simulink library "EstebanPowerLIB"  (R2013a)
settings: Solver=ode45  StartTime=0.0  StopTime=10.0  RelTol=1e-3
libraries: fl_lib x64, nesl_utility x31, elec_lib x6, dsparch4 x1
settings Model: Creator=Esteban  LastModifiedBy=Esteban

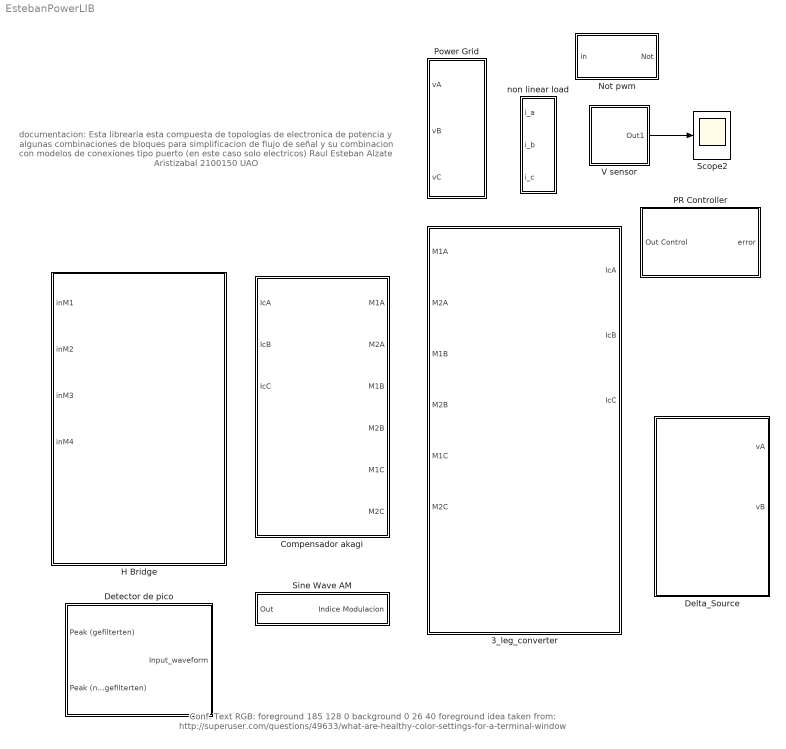
== system EstebanPowerLIB ==
  note: documentacion:
      |
      |
      | Esta librearia esta compuesta
      | de topologias de electronica de potencia
      | y algunas combinaciones de bloques
      | para simplificacion de flujo de señal
      | y su combinacion con modelos de conexiones
      | tipo puerto (en este caso solo electricos)
      |
      | Raul Esteban Alzate Aristizabal 2100150 UAO
  note: Conf. Text
      | RGB:
      | foreground 185 128 0
      | background 0 26 40
      | foreground idea taken from:
      | http://superuser.com/questions/49633/what-are-healthy-color-settings-for-a-terminal-window
  3_leg_converter : Subsystem
  Compensador akagi : Subsystem
  Delta_Source : Subsystem
  Detector de pico : Subsystem
  H Bridge : Subsystem
  Not pwm : Subsystem
  PR Controller : Subsystem
  Power Grid : Subsystem
  Scope2 : Scope
  Sine Wave AM : Subsystem
  V sensor : Subsystem
  non linear load : Subsystem
  wires:
  V sensor/1(Out1) -> Scope2/1

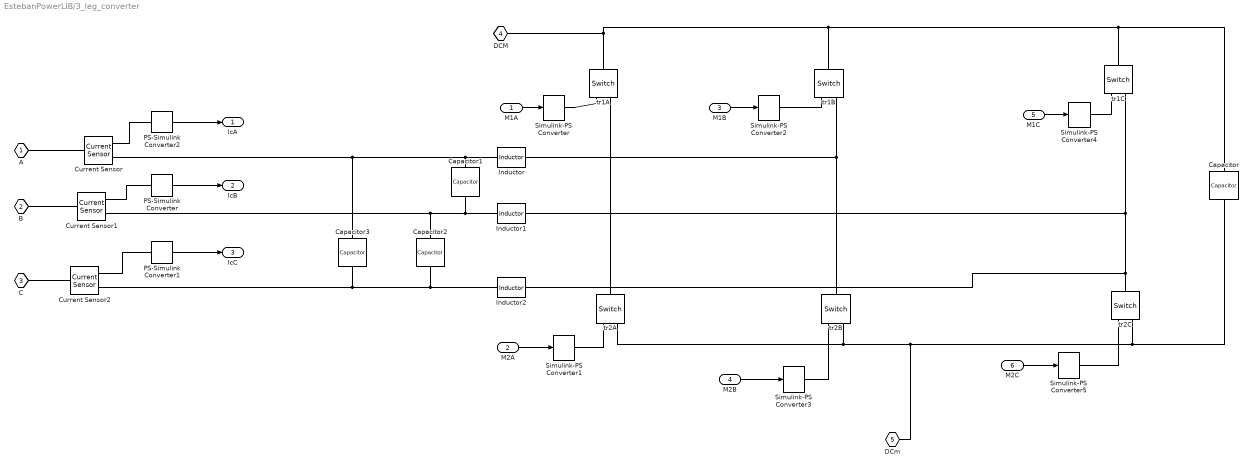
== system EstebanPowerLIB/3_leg_converter ==
  M1A : Inport
  M2A : Inport  Port=2
  M1B : Inport  Port=3
  M2B : Inport  Port=4
  M1C : Inport  Port=5
  M2C : Inport  Port=6
  Capacitor : fl_lib/Electrical/Electrical Elements/Capacitor  c=5 uF  v0=0 V  r=1e-6 Ohm  g=0 1/Ohm  i_Log=off  v_Log=off  vc_Log=off  LocalVarNames=|i|v|vc  LocalVarDescs=|i|v|Internal variable for voltage across capacitor term  LocalVarLogging=[0 0 0]
  Capacitor1 : fl_lib/Electrical/Electrical Elements/Capacitor  c=0.5 uF  v0=0 V  r=1e-6 Ohm  g=13e-8 1/Ohm  i_Log=off  v_Log=off  vc_Log=off  LocalVarNames=|i|v|vc  LocalVarDescs=|i|v|Internal variable for voltage across capacitor term  LocalVarLogging=[0 0 0]
  Capacitor2 : fl_lib/Electrical/Electrical Elements/Capacitor  c=0.5 uF  v0=0 V  r=1e-6 Ohm  g=13e-8 1/Ohm  i_Log=off  v_Log=off  vc_Log=off  LocalVarNames=|i|v|vc  LocalVarDescs=|i|v|Internal variable for voltage across capacitor term  LocalVarLogging=[0 0 0]
  Capacitor3 : fl_lib/Electrical/Electrical Elements/Capacitor  c=0.5 uF  v0=0 V  r=1e-6 Ohm  g=13e-8 1/Ohm  i_Log=off  v_Log=off  vc_Log=off  LocalVarNames=|i|v|vc  LocalVarDescs=|i|v|Internal variable for voltage across capacitor term  LocalVarLogging=[0 0 0]
  Current Sensor : fl_lib/Electrical/Electrical Sensors/Current Sensor  i1_Log=off  v1_Log=off  LocalVarNames=|i1|v1  LocalVarDescs=|i1|v1  LocalVarLogging=[0 0]
  Current Sensor1 : fl_lib/Electrical/Electrical Sensors/Current Sensor  i1_Log=off  v1_Log=off  LocalVarNames=|i1|v1  LocalVarDescs=|i1|v1  LocalVarLogging=[0 0]
  Current Sensor2 : fl_lib/Electrical/Electrical Sensors/Current Sensor  i1_Log=off  v1_Log=off  LocalVarNames=|i1|v1  LocalVarDescs=|i1|v1  LocalVarLogging=[0 0]
  Inductor : fl_lib/Electrical/Electrical Elements/Inductor  l=2.4 mH  i0=0 A  r=0.1 Ohm  g=1e-5 1/Ohm  i_Log=off  v_Log=off  i_L_Log=off  LocalVarNames=|i|v|i_L  LocalVarDescs=|i|v|Internal variable for current through inductor term  LocalVarLogging=[0 0 0]
  Inductor1 : fl_lib/Electrical/Electrical Elements/Inductor  l=2.4 mH  i0=0 A  r=0.1 Ohm  g=1e-5 1/Ohm  i_Log=off  v_Log=off  i_L_Log=off  LocalVarNames=|i|v|i_L  LocalVarDescs=|i|v|Internal variable for current through inductor term  LocalVarLogging=[0 0 0]
  Inductor2 : fl_lib/Electrical/Electrical Elements/Inductor  l=2.4 mH  i0=0 A  r=0.1 Ohm  g=1e-5 1/Ohm  i_Log=off  v_Log=off  i_L_Log=off  LocalVarNames=|i|v|i_L  LocalVarDescs=|i|v|Internal variable for current through inductor term  LocalVarLogging=[0 0 0]
  PS-Simulink Converter : nesl_utility/PS-Simulink Converter  PhysicalDomain=network_engine_domain  SubClassName=ps_output  LeftPortType=input  RightPortType=output  PseudoPeriodic=off  Frequencies=[]  Unit=1  AffineConversion=off
  PS-Simulink Converter1 : nesl_utility/PS-Simulink Converter  PhysicalDomain=network_engine_domain  SubClassName=ps_output  LeftPortType=input  RightPortType=output  PseudoPeriodic=off  Frequencies=[]  Unit=1  AffineConversion=off
  PS-Simulink Converter2 : nesl_utility/PS-Simulink Converter  PhysicalDomain=network_engine_domain  SubClassName=ps_output  LeftPortType=input  RightPortType=output  PseudoPeriodic=off  Frequencies=[]  Unit=1  AffineConversion=off
  Simulink-PS Converter{,1..5} (6 alike) : nesl_utility/Simulink-PS Converter  PhysicalDomain=network_engine_domain  SubClassName=ps_input  LeftPortType=input  RightPortType=output  PseudoPeriodic=off  Frequencies=[]  NoiseDistribution=none  NoiseParameters=[]  Unit=1  AffineConversion=off  InputFiltering=off  SimscapeFilterOrder=1  InputFilterTimeConstant=0.001  UdotUserProvided=1
  tr1A : fl_lib/Electrical/Electrical Elements/Switch  R_closed=0.01 Ohm  G_open=1e-8 1/Ohm  Threshold=10  i_Log=off  v_Log=off  LocalVarNames=|i|v  LocalVarDescs=|i|v  LocalVarLogging=[0 0]
  tr1B : fl_lib/Electrical/Electrical Elements/Switch  R_closed=0.01 Ohm  G_open=1e-8 1/Ohm  Threshold=10  i_Log=off  v_Log=off  LocalVarNames=|i|v  LocalVarDescs=|i|v  LocalVarLogging=[0 0]
  tr1C : fl_lib/Electrical/Electrical Elements/Switch  R_closed=0.01 Ohm  G_open=1e-8 1/Ohm  Threshold=10  i_Log=off  v_Log=off  LocalVarNames=|i|v  LocalVarDescs=|i|v  LocalVarLogging=[0 0]
  tr2A : fl_lib/Electrical/Electrical Elements/Switch  R_closed=0.01 Ohm  G_open=1e-8 1/Ohm  Threshold=10  i_Log=off  v_Log=off  LocalVarNames=|i|v  LocalVarDescs=|i|v  LocalVarLogging=[0 0]
  tr2B : fl_lib/Electrical/Electrical Elements/Switch  R_closed=0.01 Ohm  G_open=1e-8 1/Ohm  Threshold=10  i_Log=off  v_Log=off  LocalVarNames=|i|v  LocalVarDescs=|i|v  LocalVarLogging=[0 0]
  tr2C : fl_lib/Electrical/Electrical Elements/Switch  R_closed=0.01 Ohm  G_open=1e-8 1/Ohm  Threshold=10  i_Log=off  v_Log=off  LocalVarNames=|i|v  LocalVarDescs=|i|v  LocalVarLogging=[0 0]
  A : PMIOPort  Port=1  Side=Right
  B : PMIOPort  Port=2  Side=Right
  C : PMIOPort  Port=3  Side=Right
  DCM : PMIOPort  Port=4  Side=Left
  DCm : PMIOPort  Port=5  Side=Left
  IcA : Outport
  IcB : Outport  Port=2
  IcC : Outport  Port=3
  wires:
  M2C/1 -> Simulink-PS Converter5/1
  M1C/1 -> Simulink-PS Converter4/1
  M2B/1 -> Simulink-PS Converter3/1
  M1B/1 -> Simulink-PS Converter2/1
  M2A/1 -> Simulink-PS Converter1/1
  M1A/1 -> Simulink-PS Converter/1
  PS-Simulink Converter2/1 -> IcA/1
  PS-Simulink Converter/1 -> IcB/1
  PS-Simulink Converter1/1 -> IcC/1
  connections:
  Simulink-PS Converter3/RConn1 -- tr2B/RConn1
  Simulink-PS Converter4/RConn1 -- tr1C/RConn1
  Simulink-PS Converter/RConn1 -- tr1A/RConn1
  Simulink-PS Converter5/RConn1 -- tr2C/RConn1
  tr2A/RConn1 -- Simulink-PS Converter1/RConn1
  tr2C/RConn2 -- DCm/RConn1 -- tr2A/RConn2 -- tr2B/RConn2 -- Capacitor/RConn1
  tr1A/RConn2 -- tr2A/LConn1
  tr1B/RConn2 -- Inductor/RConn1 -- tr2B/LConn1
  Capacitor/LConn1 -- tr1C/LConn1 -- DCM/RConn1 -- tr1A/LConn1 -- tr1B/LConn1
  tr1C/RConn2 -- Inductor1/RConn1 -- Inductor2/RConn1 -- tr2C/LConn1
  tr1B/RConn1 -- Simulink-PS Converter2/RConn1
  Capacitor1/LConn1 -- Inductor/LConn1 -- Capacitor3/LConn1 -- Current Sensor/RConn2
  Capacitor1/RConn1 -- Inductor1/LConn1 -- Capacitor2/LConn1 -- Current Sensor1/RConn2
  Capacitor2/RConn1 -- Inductor2/LConn1 -- Current Sensor2/RConn2 -- Capacitor3/RConn1
  Current Sensor1/RConn1 -- PS-Simulink Converter/LConn1
  Current Sensor/RConn1 -- PS-Simulink Converter2/LConn1
  Current Sensor2/RConn1 -- PS-Simulink Converter1/LConn1
  B/RConn1 -- Current Sensor1/LConn1
  A/RConn1 -- Current Sensor/LConn1
  Current Sensor2/LConn1 -- C/RConn1

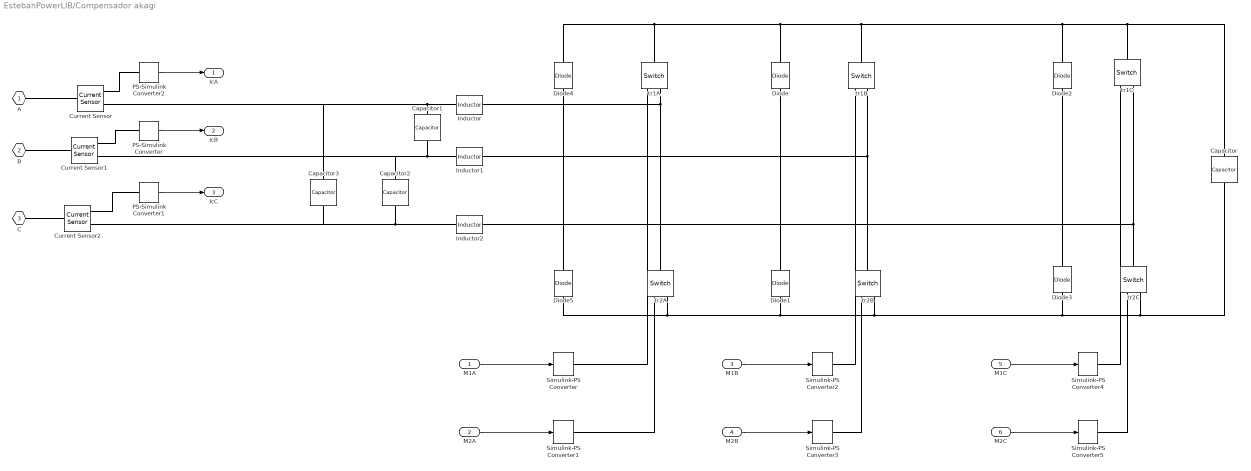
== system EstebanPowerLIB/Compensador akagi ==
  M1A : Inport
  M2A : Inport  Port=2
  M1B : Inport  Port=3
  M2B : Inport  Port=4
  M1C : Inport  Port=5
  M2C : Inport  Port=6
  Capacitor : fl_lib/Electrical/Electrical Elements/Capacitor  c=5 uF  v0=0 V  r=1e-6 Ohm  g=0 1/Ohm  i_Log=off  v_Log=off  vc_Log=off  LocalVarNames=|i|v|vc  LocalVarDescs=|i|v|Internal variable for voltage across capacitor term  LocalVarLogging=[0 0 0]
  Capacitor1 : fl_lib/Electrical/Electrical Elements/Capacitor  c=0.5 uF  v0=0 V  r=1e-6 Ohm  g=0 1/Ohm  i_Log=off  v_Log=off  vc_Log=off  LocalVarNames=|i|v|vc  LocalVarDescs=|i|v|Internal variable for voltage across capacitor term  LocalVarLogging=[0 0 0]
  Capacitor2 : fl_lib/Electrical/Electrical Elements/Capacitor  c=0.5 uF  v0=0 V  r=1e-6 Ohm  g=0 1/Ohm  i_Log=off  v_Log=off  vc_Log=off  LocalVarNames=|i|v|vc  LocalVarDescs=|i|v|Internal variable for voltage across capacitor term  LocalVarLogging=[0 0 0]
  Capacitor3 : fl_lib/Electrical/Electrical Elements/Capacitor  c=0.5 uF  v0=0 V  r=1e-6 Ohm  g=0 1/Ohm  i_Log=off  v_Log=off  vc_Log=off  LocalVarNames=|i|v|vc  LocalVarDescs=|i|v|Internal variable for voltage across capacitor term  LocalVarLogging=[0 0 0]
  Current Sensor : fl_lib/Electrical/Electrical Sensors/Current Sensor  i1_Log=off  v1_Log=off  LocalVarNames=|i1|v1  LocalVarDescs=|i1|v1  LocalVarLogging=[0 0]
  Current Sensor1 : fl_lib/Electrical/Electrical Sensors/Current Sensor  i1_Log=off  v1_Log=off  LocalVarNames=|i1|v1  LocalVarDescs=|i1|v1  LocalVarLogging=[0 0]
  Current Sensor2 : fl_lib/Electrical/Electrical Sensors/Current Sensor  i1_Log=off  v1_Log=off  LocalVarNames=|i1|v1  LocalVarDescs=|i1|v1  LocalVarLogging=[0 0]
  Diode{,1..5} (6 alike) : fl_lib/Electrical/Electrical Elements/Diode  Vf=0.6 V  Ron=0.3 Ohm  Goff=1e-8 1/Ohm  i_Log=off  v_Log=off  LocalVarNames=|i|v  LocalVarDescs=|i|v  LocalVarLogging=[0 0]
  Inductor : fl_lib/Electrical/Electrical Elements/Inductor  l=2.4 mH  i0=0 A  r=0.1 Ohm  g=1e-9 1/Ohm  i_Log=off  v_Log=off  i_L_Log=off  LocalVarNames=|i|v|i_L  LocalVarDescs=|i|v|Internal variable for current through inductor term  LocalVarLogging=[0 0 0]
  Inductor1 : fl_lib/Electrical/Electrical Elements/Inductor  l=2.4 mH  i0=0 A  r=0.1 Ohm  g=1e-9 1/Ohm  i_Log=off  v_Log=off  i_L_Log=off  LocalVarNames=|i|v|i_L  LocalVarDescs=|i|v|Internal variable for current through inductor term  LocalVarLogging=[0 0 0]
  Inductor2 : fl_lib/Electrical/Electrical Elements/Inductor  l=2.4 mH  i0=0 A  r=0.1 Ohm  g=1e-9 1/Ohm  i_Log=off  v_Log=off  i_L_Log=off  LocalVarNames=|i|v|i_L  LocalVarDescs=|i|v|Internal variable for current through inductor term  LocalVarLogging=[0 0 0]
  PS-Simulink Converter : nesl_utility/PS-Simulink Converter  PhysicalDomain=network_engine_domain  SubClassName=ps_output  LeftPortType=input  RightPortType=output  PseudoPeriodic=off  Frequencies=[]  Unit=1  AffineConversion=off
  PS-Simulink Converter1 : nesl_utility/PS-Simulink Converter  PhysicalDomain=network_engine_domain  SubClassName=ps_output  LeftPortType=input  RightPortType=output  PseudoPeriodic=off  Frequencies=[]  Unit=1  AffineConversion=off
  PS-Simulink Converter2 : nesl_utility/PS-Simulink Converter  PhysicalDomain=network_engine_domain  SubClassName=ps_output  LeftPortType=input  RightPortType=output  PseudoPeriodic=off  Frequencies=[]  Unit=1  AffineConversion=off
  Simulink-PS Converter{,1..5} (6 alike) : nesl_utility/Simulink-PS Converter  PhysicalDomain=network_engine_domain  SubClassName=ps_input  LeftPortType=input  RightPortType=output  PseudoPeriodic=off  Frequencies=[]  NoiseDistribution=none  NoiseParameters=[]  Unit=1  AffineConversion=off  InputFiltering=off  SimscapeFilterOrder=1  InputFilterTimeConstant=0.001  UdotUserProvided=1
  tr1A : fl_lib/Electrical/Electrical Elements/Switch  R_closed=0.01 Ohm  G_open=1e-8 1/Ohm  Threshold=10  i_Log=off  v_Log=off  LocalVarNames=|i|v  LocalVarDescs=|i|v  LocalVarLogging=[0 0]
  tr1B : fl_lib/Electrical/Electrical Elements/Switch  R_closed=0.01 Ohm  G_open=1e-8 1/Ohm  Threshold=10  i_Log=off  v_Log=off  LocalVarNames=|i|v  LocalVarDescs=|i|v  LocalVarLogging=[0 0]
  tr1C : fl_lib/Electrical/Electrical Elements/Switch  R_closed=0.01 Ohm  G_open=1e-8 1/Ohm  Threshold=10  i_Log=off  v_Log=off  LocalVarNames=|i|v  LocalVarDescs=|i|v  LocalVarLogging=[0 0]
  tr2A : fl_lib/Electrical/Electrical Elements/Switch  R_closed=0.01 Ohm  G_open=1e-8 1/Ohm  Threshold=10  i_Log=off  v_Log=off  LocalVarNames=|i|v  LocalVarDescs=|i|v  LocalVarLogging=[0 0]
  tr2B : fl_lib/Electrical/Electrical Elements/Switch  R_closed=0.01 Ohm  G_open=1e-8 1/Ohm  Threshold=10  i_Log=off  v_Log=off  LocalVarNames=|i|v  LocalVarDescs=|i|v  LocalVarLogging=[0 0]
  tr2C : fl_lib/Electrical/Electrical Elements/Switch  R_closed=0.01 Ohm  G_open=1e-8 1/Ohm  Threshold=10  i_Log=off  v_Log=off  LocalVarNames=|i|v  LocalVarDescs=|i|v  LocalVarLogging=[0 0]
  A : PMIOPort  Port=1  Side=Right
  B : PMIOPort  Port=2  Side=Right
  C : PMIOPort  Port=3  Side=Right
  IcA : Outport
  IcB : Outport  Port=2
  IcC : Outport  Port=3
  wires:
  M1A/1 -> Simulink-PS Converter/1
  M2A/1 -> Simulink-PS Converter1/1
  M1B/1 -> Simulink-PS Converter2/1
  M2B/1 -> Simulink-PS Converter3/1
  M1C/1 -> Simulink-PS Converter4/1
  M2C/1 -> Simulink-PS Converter5/1
  PS-Simulink Converter2/1 -> IcA/1
  PS-Simulink Converter/1 -> IcB/1
  PS-Simulink Converter1/1 -> IcC/1
  connections:
  tr2A/RConn2 -- Diode1/LConn1 -- tr2B/RConn2 -- Diode3/LConn1 -- Capacitor/RConn1 -- tr2C/RConn2 -- Diode5/LConn1
  tr1A/RConn2 -- tr2A/LConn1 -- Inductor/RConn1 -- Diode5/RConn1 -- Diode4/LConn1
  tr1B/RConn2 -- Inductor1/RConn1 -- Diode/LConn1 -- Diode1/RConn1 -- tr2B/LConn1
  tr1C/LConn1 -- Diode2/RConn1 -- Diode/RConn1 -- Diode4/RConn1 -- tr1A/LConn1 -- tr1B/LConn1 -- Capacitor/LConn1
  tr1C/RConn2 -- Inductor2/RConn1 -- Diode3/RConn1 -- Diode2/LConn1 -- tr2C/LConn1
  Inductor/LConn1 -- Capacitor3/LConn1 -- Current Sensor/RConn2 -- Capacitor1/LConn1
  Inductor1/LConn1 -- Capacitor2/LConn1 -- Current Sensor1/RConn2 -- Capacitor1/RConn1
  Inductor2/LConn1 -- Current Sensor2/RConn2 -- Capacitor3/RConn1 -- Capacitor2/RConn1
  Simulink-PS Converter/RConn1 -- tr1A/RConn1
  Simulink-PS Converter1/RConn1 -- tr2A/RConn1
  Simulink-PS Converter3/RConn1 -- tr2B/RConn1
  Simulink-PS Converter2/RConn1 -- tr1B/RConn1
  Simulink-PS Converter4/RConn1 -- tr1C/RConn1
  Simulink-PS Converter5/RConn1 -- tr2C/RConn1
  A/RConn1 -- Current Sensor/LConn1
  B/RConn1 -- Current Sensor1/LConn1
  Current Sensor2/LConn1 -- C/RConn1
  Current Sensor2/RConn1 -- PS-Simulink Converter1/LConn1
  Current Sensor1/RConn1 -- PS-Simulink Converter/LConn1
  Current Sensor/RConn1 -- PS-Simulink Converter2/LConn1

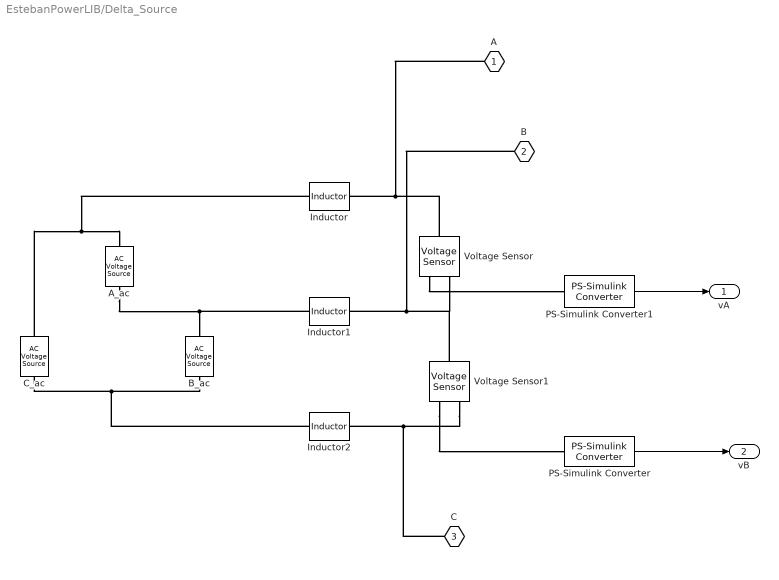
== system EstebanPowerLIB/Delta_Source ==
  A_ac : fl_lib/Electrical/Electrical Sources/AC Voltage Source  amp=170 V  shift=0 deg  frequency=60 Hz  omega=0 rad/s  i_Log=off  v_Log=off  LocalVarNames=|i|v  LocalVarDescs=|i|v  LocalVarLogging=[0 0]
  B_ac : fl_lib/Electrical/Electrical Sources/AC Voltage Source  amp=170 V  shift=-120 deg  frequency=60 Hz  omega=0 rad/s  i_Log=off  v_Log=off  LocalVarNames=|i|v  LocalVarDescs=|i|v  LocalVarLogging=[0 0]
  C_ac : fl_lib/Electrical/Electrical Sources/AC Voltage Source  amp=170 V  shift=120 deg  frequency=60 Hz  omega=0 rad/s  i_Log=off  v_Log=off  LocalVarNames=|i|v  LocalVarDescs=|i|v  LocalVarLogging=[0 0]
  Inductor : fl_lib/Electrical/Electrical Elements/Inductor  l=2 mH  i0=0 A  r=0.2 Ohm  g=1e-4 1/Ohm  i_Log=off  v_Log=off  i_L_Log=off  LocalVarNames=|i|v|i_L  LocalVarDescs=|i|v|Internal variable for current through inductor term  LocalVarLogging=[0 0 0]
  Inductor1 : fl_lib/Electrical/Electrical Elements/Inductor  l=2 mH  i0=0 A  r=0.2 Ohm  g=1e-4 1/Ohm  i_Log=off  v_Log=off  i_L_Log=off  LocalVarNames=|i|v|i_L  LocalVarDescs=|i|v|Internal variable for current through inductor term  LocalVarLogging=[0 0 0]
  Inductor2 : fl_lib/Electrical/Electrical Elements/Inductor  l=2 mH  i0=0 A  r=0.1 Ohm  g=1e-4 1/Ohm  i_Log=off  v_Log=off  i_L_Log=off  LocalVarNames=|i|v|i_L  LocalVarDescs=|i|v|Internal variable for current through inductor term  LocalVarLogging=[0 0 0]
  PS-Simulink Converter : nesl_utility/PS-Simulink Converter  PhysicalDomain=network_engine_domain  SubClassName=ps_output  LeftPortType=input  RightPortType=output  PseudoPeriodic=off  Frequencies=[]  Unit=1  AffineConversion=off
  PS-Simulink Converter1 : nesl_utility/PS-Simulink Converter  PhysicalDomain=network_engine_domain  SubClassName=ps_output  LeftPortType=input  RightPortType=output  PseudoPeriodic=off  Frequencies=[]  Unit=1  AffineConversion=off
  Voltage Sensor : fl_lib/Electrical/Electrical Sensors/Voltage Sensor  i1_Log=off  v1_Log=off  LocalVarNames=|i1|v1  LocalVarDescs=|i1|v1  LocalVarLogging=[0 0]
  Voltage Sensor1 : fl_lib/Electrical/Electrical Sensors/Voltage Sensor  i1_Log=off  v1_Log=off  LocalVarNames=|i1|v1  LocalVarDescs=|i1|v1  LocalVarLogging=[0 0]
  A : PMIOPort  Port=1  Side=Left
  B : PMIOPort  Port=2  Side=Right
  C : PMIOPort  Port=3  Side=Left
  vA : Outport
  vB : Outport  Port=2
  wires:
  PS-Simulink Converter1/1 -> vA/1
  PS-Simulink Converter/1 -> vB/1
  connections:
  Voltage Sensor/RConn1 -- PS-Simulink Converter1/LConn1
  Inductor2/LConn1 -- B_ac/RConn1 -- C_ac/RConn1
  Voltage Sensor1/RConn1 -- PS-Simulink Converter/LConn1
  C/RConn1 -- Voltage Sensor1/RConn2 -- Inductor2/RConn1
  Inductor1/LConn1 -- A_ac/RConn1 -- B_ac/LConn1
  A/RConn1 -- Voltage Sensor/LConn1 -- Inductor/RConn1
  Inductor/LConn1 -- C_ac/LConn1 -- A_ac/LConn1
  B/RConn1 -- Voltage Sensor1/LConn1 -- Voltage Sensor/RConn2 -- Inductor1/RConn1

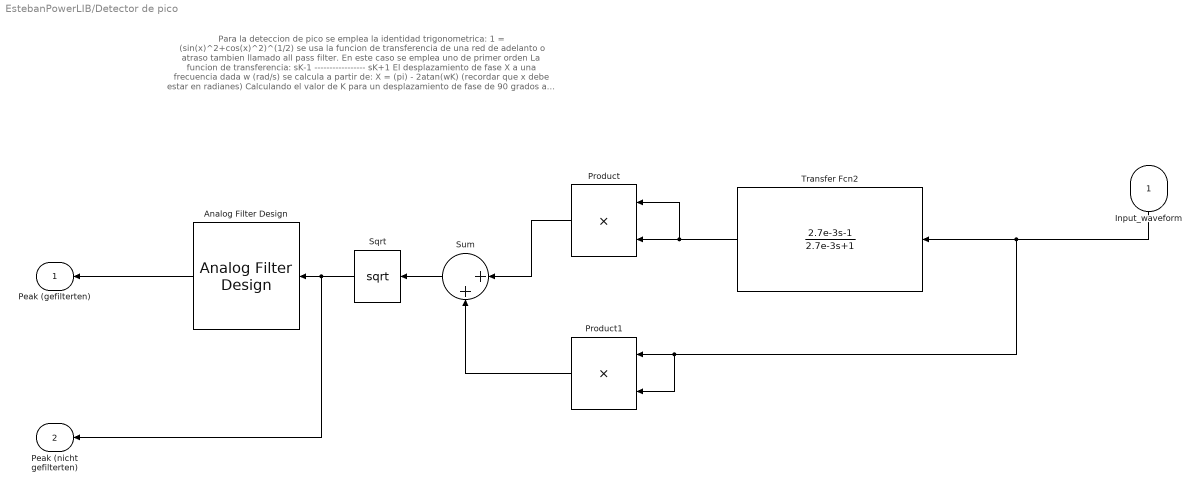
== system EstebanPowerLIB/Detector de pico ==
  note: Para la deteccion de pico se emplea la identidad trigonometrica:
      | 1 = (sin(x)^2+cos(x)^2)^(1/2)
      | se usa la funcion de transferencia de una red de adelanto o atraso
      | tambien llamado all pass filter. En este caso se emplea uno de primer orden
      | La funcion de transferencia:
      | sK-1
      | -----------------
      | sK+1
      | El desplazamiento de fase X a una frecuencia dada w (rad/s) se calcula a partir de:
      | X = (pi) - 2atan(wK)
      | (recordar que x debe estar en radianes)
      | Calculando el valor de K para un desplazamiento de fase de 90 grados
      | a 60 Hz se logra obtener de la señal su "coseno".
      | seguido de esto solo basta con elevarlas ambas al cuadrado y sumarlas.
      | finalmente la raiz cuadrada es el valor pico de la señal y este metodo es aplicable durante
      | todo el periodo de la forma de onda. para reducir el ruido por conmutacion se agrega un  filtro
      | a la salida del detector. este filtro efectivamente permite obtener una señal mas limpia
      | pero reduce la velocidad de reaccion del detector de pico. Asi como esta configurado se puede
      | esperar una desviacion de no mas que 1ms.
  Input_waveform : Inport
  Analog Filter Design : dsparch4/Analog Filter Design  method=Bessel  filttype=Lowpass  N=8  Wlo=4900*2*pi  Whi=80  Rp=2  Rs=40
  Product : Product
  Product1 : Product
  Sqrt : Sqrt  SaturateOnIntegerOverflow=on
  Sum : Sum  Inputs=|++
  Transfer Fcn2 : TransferFcn  Numerator=[2.7e-3 -1]  Denominator=[2.7e-3 +1]
  Peak (gefilterten) : Outport
  Peak (nicht gefilterten) : Outport  Port=2
  wires:
  Transfer Fcn2/1 -> Product/2, Product/1
  Sum/1 -> Sqrt/1
  Sqrt/1 -> Analog Filter Design/1, Peak (nicht gefilterten)/1
  Product/1 -> Sum/1
  Product1/1 -> Sum/2
  Analog Filter Design/1 -> Peak (gefilterten)/1
  Input_waveform/1 -> Transfer Fcn2/1, Product1/1, Product1/2

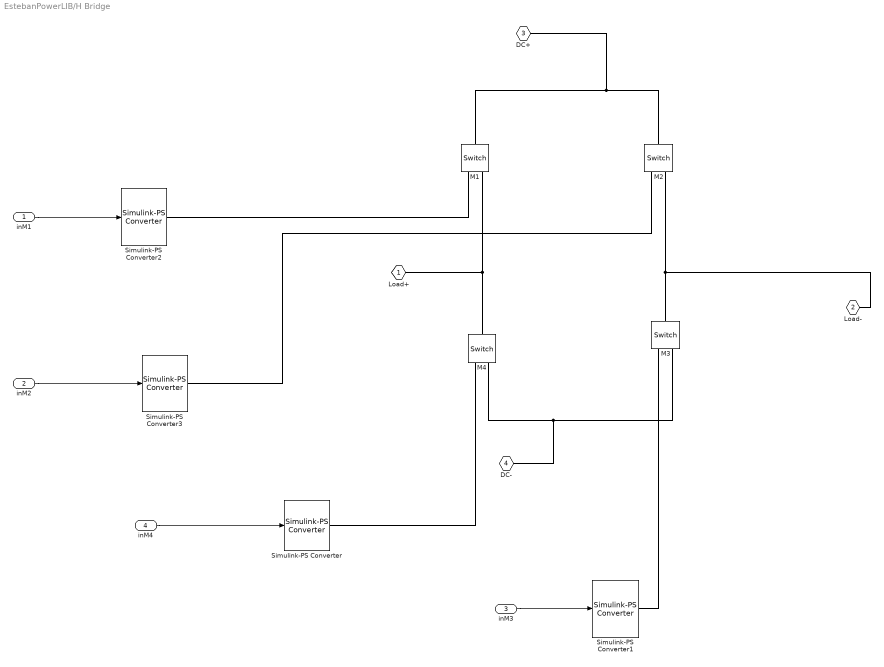
== system EstebanPowerLIB/H Bridge ==
  "inM1 " : Inport
  inM2 : Inport  Port=2
  inM3 : Inport  Port=3
  inM4 : Inport  Port=4
  M{1..4} (4 alike) : fl_lib/Electrical/Electrical Elements/Switch  R_closed=0.01 Ohm  G_open=1e-8 1/Ohm  Threshold=10  i_Log=off  v_Log=off  LocalVarNames=|i|v  LocalVarDescs=|i|v  LocalVarLogging=[0 0]
  Simulink-PS Converter{,1..3} (4 alike) : nesl_utility/Simulink-PS Converter  PhysicalDomain=network_engine_domain  SubClassName=ps_input  LeftPortType=input  RightPortType=output  PseudoPeriodic=off  Frequencies=[]  NoiseDistribution=none  NoiseParameters=[]  Unit=1  AffineConversion=off  InputFiltering=off  SimscapeFilterOrder=1  InputFilterTimeConstant=0.001  UdotUserProvided=1
  Load+ : PMIOPort  Port=1  Side=Right
  Load- : PMIOPort  Port=2  Side=Right
  DC+ : PMIOPort  Port=3  Side=Left
  DC- : PMIOPort  Port=4  Side=Left
  wires:
  "inM1 "/1 -> Simulink-PS Converter2/1
  inM2/1 -> Simulink-PS Converter3/1
  inM3/1 -> Simulink-PS Converter1/1
  inM4/1 -> Simulink-PS Converter/1
  connections:
  Simulink-PS Converter1/RConn1 -- M3/RConn1
  Simulink-PS Converter/RConn1 -- M4/RConn1
  Simulink-PS Converter3/RConn1 -- M2/RConn1
  Simulink-PS Converter2/RConn1 -- M1/RConn1
  M2/LConn1 -- DC+/RConn1 -- M1/LConn1
  M3/RConn2 -- DC-/RConn1 -- M4/RConn2
  M2/RConn2 -- M3/LConn1 -- Load-/RConn1
  M1/RConn2 -- Load+/RConn1 -- M4/LConn1

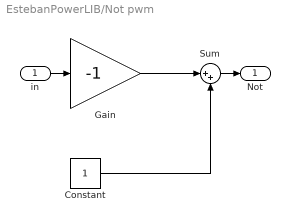
== system EstebanPowerLIB/Not pwm ==
  in : Inport
  Constant : Constant
  Gain : Gain  Gain=-1
  Sum : Sum  Inputs=|++
  Not : Outport
  wires:
  Sum/1 -> Not/1
  in/1 -> Gain/1
  Constant/1 -> Sum/2
  Gain/1 -> Sum/1

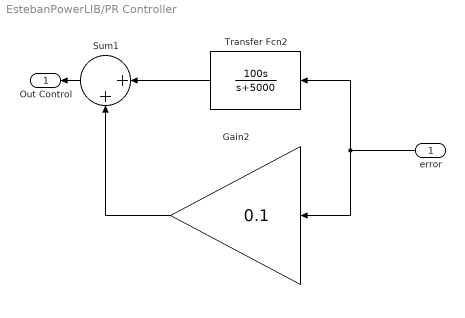
== system EstebanPowerLIB/PR Controller ==
  error : Inport
  Gain2 : Gain  Gain=0.1
  Sum1 : Sum  Inputs=|++
  Transfer Fcn2 : TransferFcn  Numerator=[100 0]  Denominator=[1 5000]
  Out Control : Outport
  wires:
  Gain2/1 -> Sum1/2
  Transfer Fcn2/1 -> Sum1/1
  Sum1/1 -> Out Control/1
  error/1 -> Transfer Fcn2/1, Gain2/1

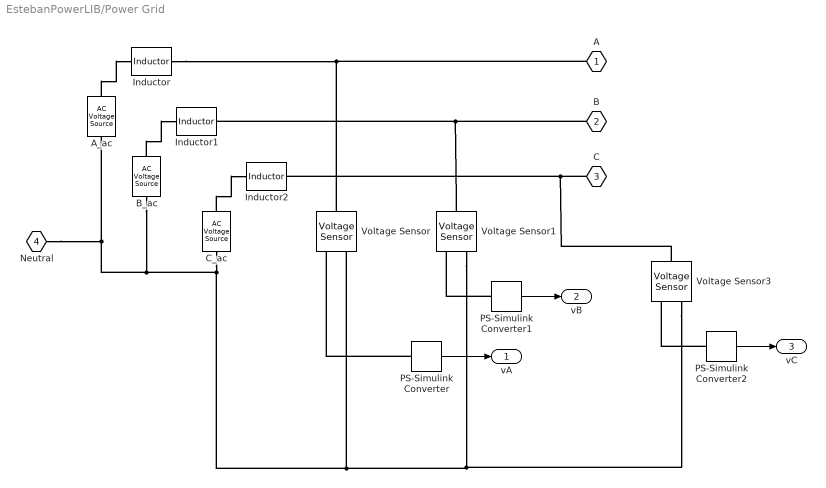
== system EstebanPowerLIB/Power Grid ==
  A_ac : fl_lib/Electrical/Electrical Sources/AC Voltage Source  amp=170 V  shift=0 deg  frequency=60 Hz  omega=0 rad/s  i_Log=off  v_Log=off  LocalVarNames=|i|v  LocalVarDescs=|i|v  LocalVarLogging=[0 0]
  B_ac : fl_lib/Electrical/Electrical Sources/AC Voltage Source  amp=170 V  shift=-120 deg  frequency=60 Hz  omega=0 rad/s  i_Log=off  v_Log=off  LocalVarNames=|i|v  LocalVarDescs=|i|v  LocalVarLogging=[0 0]
  C_ac : fl_lib/Electrical/Electrical Sources/AC Voltage Source  amp=170 V  shift=120 deg  frequency=60 Hz  omega=0 rad/s  i_Log=off  v_Log=off  LocalVarNames=|i|v  LocalVarDescs=|i|v  LocalVarLogging=[0 0]
  Inductor : fl_lib/Electrical/Electrical Elements/Inductor  l=2 mH  i0=0 A  r=0.2 Ohm  g=1e-4 1/Ohm  i_Log=off  v_Log=off  i_L_Log=off  LocalVarNames=|i|v|i_L  LocalVarDescs=|i|v|Internal variable for current through inductor term  LocalVarLogging=[0 0 0]
  Inductor1 : fl_lib/Electrical/Electrical Elements/Inductor  l=2 mH  i0=0 A  r=0.2 Ohm  g=1e-4 1/Ohm  i_Log=off  v_Log=off  i_L_Log=off  LocalVarNames=|i|v|i_L  LocalVarDescs=|i|v|Internal variable for current through inductor term  LocalVarLogging=[0 0 0]
  Inductor2 : fl_lib/Electrical/Electrical Elements/Inductor  l=2 mH  i0=0 A  r=0.1 Ohm  g=1e-4 1/Ohm  i_Log=off  v_Log=off  i_L_Log=off  LocalVarNames=|i|v|i_L  LocalVarDescs=|i|v|Internal variable for current through inductor term  LocalVarLogging=[0 0 0]
  PS-Simulink Converter : nesl_utility/PS-Simulink Converter  PhysicalDomain=network_engine_domain  SubClassName=ps_output  LeftPortType=input  RightPortType=output  PseudoPeriodic=off  Frequencies=[]  Unit=1  AffineConversion=off
  PS-Simulink Converter1 : nesl_utility/PS-Simulink Converter  PhysicalDomain=network_engine_domain  SubClassName=ps_output  LeftPortType=input  RightPortType=output  PseudoPeriodic=off  Frequencies=[]  Unit=1  AffineConversion=off
  PS-Simulink Converter2 : nesl_utility/PS-Simulink Converter  PhysicalDomain=network_engine_domain  SubClassName=ps_output  LeftPortType=input  RightPortType=output  PseudoPeriodic=off  Frequencies=[]  Unit=1  AffineConversion=off
  Voltage Sensor : fl_lib/Electrical/Electrical Sensors/Voltage Sensor  i1_Log=off  v1_Log=off  LocalVarNames=|i1|v1  LocalVarDescs=|i1|v1  LocalVarLogging=[0 0]
  Voltage Sensor1 : fl_lib/Electrical/Electrical Sensors/Voltage Sensor  i1_Log=off  v1_Log=off  LocalVarNames=|i1|v1  LocalVarDescs=|i1|v1  LocalVarLogging=[0 0]
  Voltage Sensor3 : fl_lib/Electrical/Electrical Sensors/Voltage Sensor  i1_Log=off  v1_Log=off  LocalVarNames=|i1|v1  LocalVarDescs=|i1|v1  LocalVarLogging=[0 0]
  A : PMIOPort  Port=1  Side=Left
  B : PMIOPort  Port=2  Side=Left
  C : PMIOPort  Port=3  Side=Left
  Neutral : PMIOPort  Port=4  Side=Left
  vA : Outport
  vB : Outport  Port=2
  vC : Outport  Port=3
  wires:
  PS-Simulink Converter/1 -> vA/1
  PS-Simulink Converter1/1 -> vB/1
  PS-Simulink Converter2/1 -> vC/1
  connections:
  C_ac/LConn1 -- Inductor2/LConn1
  A_ac/LConn1 -- Inductor/LConn1
  B_ac/LConn1 -- Inductor1/LConn1
  B/RConn1 -- Voltage Sensor1/LConn1 -- Inductor1/RConn1
  PS-Simulink Converter/LConn1 -- Voltage Sensor/RConn1
  C/RConn1 -- Voltage Sensor3/LConn1 -- Inductor2/RConn1
  Inductor/RConn1 -- A/RConn1 -- Voltage Sensor/LConn1
  A_ac/RConn1 -- Neutral/RConn1 -- Voltage Sensor3/RConn2 -- Voltage Sensor1/RConn2 -- Voltage Sensor/RConn2 -- C_ac/RConn1 -- B_ac/RConn1
  PS-Simulink Converter1/LConn1 -- Voltage Sensor1/RConn1
  PS-Simulink Converter2/LConn1 -- Voltage Sensor3/RConn1

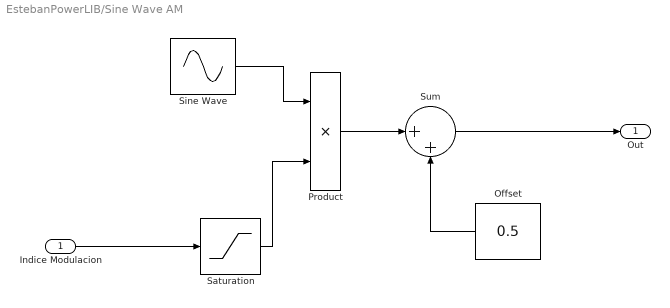
== system EstebanPowerLIB/Sine Wave AM ==
  Indice Modulacion : Inport
  Offset : Constant  Value=0.5
  Product : Product
  Saturation : Saturate  UpperLimit=1  LowerLimit=0
  Sine Wave : Sin  Amplitude=0.5  Frequency=60*2*pi  SampleTime=0
  Sum : Sum  Inputs=|++
  Out : Outport
  wires:
  Indice Modulacion/1 -> Saturation/1
  Saturation/1 -> Product/2
  Sum/1 -> Out/1
  Offset/1 -> Sum/2
  Sine Wave/1 -> Product/1
  Product/1 -> Sum/1

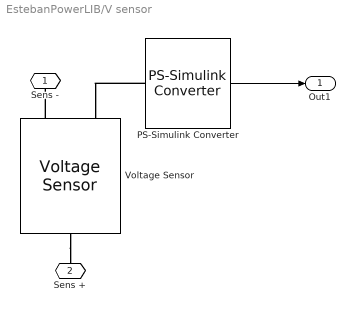
== system EstebanPowerLIB/V sensor ==
  PS-Simulink Converter : nesl_utility/PS-Simulink Converter  PhysicalDomain=network_engine_domain  SubClassName=ps_output  LeftPortType=input  RightPortType=output  PseudoPeriodic=off  Frequencies=[]  Unit=1  AffineConversion=off
  Voltage Sensor : fl_lib/Electrical/Electrical Sensors/Voltage Sensor  i1_Log=off  v1_Log=off  LocalVarNames=|i1|v1  LocalVarDescs=|i1|v1  LocalVarLogging=[0 0]
  Sens - : PMIOPort  Port=1  Side=Left
  Sens + : PMIOPort  Port=2  Side=Left
  Out1 : Outport
  wires:
  PS-Simulink Converter/1 -> Out1/1
  connections:
  Voltage Sensor/LConn1 -- Sens +/RConn1
  Voltage Sensor/RConn2 -- Sens -/RConn1
  PS-Simulink Converter/LConn1 -- Voltage Sensor/RConn1

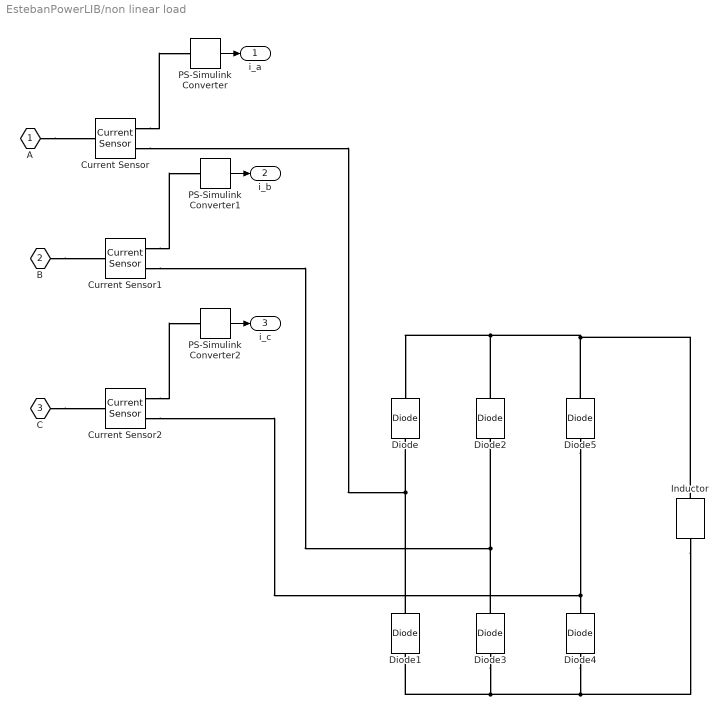
== system EstebanPowerLIB/non linear load ==
  Current Sensor : fl_lib/Electrical/Electrical Sensors/Current Sensor  i1_Log=off  v1_Log=off  LocalVarNames=|i1|v1  LocalVarDescs=|i1|v1  LocalVarLogging=[0 0]
  Current Sensor1 : fl_lib/Electrical/Electrical Sensors/Current Sensor  i1_Log=off  v1_Log=off  LocalVarNames=|i1|v1  LocalVarDescs=|i1|v1  LocalVarLogging=[0 0]
  Current Sensor2 : fl_lib/Electrical/Electrical Sensors/Current Sensor  i1_Log=off  v1_Log=off  LocalVarNames=|i1|v1  LocalVarDescs=|i1|v1  LocalVarLogging=[0 0]
  Diode{,1..5} (6 alike) : elec_lib/Semiconductor Devices/Diode  ModelType=1  Vf=0.6 V  Ron=0.3 Ohm  Goff=1e-8 S  Rz=0.3 Ohm  Vz=50 V  C_PWL=5 pF  prmExp=1  I12=[ 0.0137 0.545 ] A  V12=[ 0.6 0.7 ] V  I1=0.0137 A  V1=0.6 V  RS=0.01 Ohm  IS=1e-12 A  Tmeas=25 C  ec=1  BV=Inf V  C_param=1  CJ0=5 pF  VJ=1 V  Mgrad=0.5  Vvec=[ 0.1 10 100 ] V  Cvec=[ 3.5 1 0.4 ] pF  FC=0.5  Q_param=1  Irrm=-7.15 A  iF=4 A  didt=-750 A/us  trr=115 ns  TT=50 ns  tau=100 ns  T_param=1  IS_T2=1.25e-7 A  I1_T2=0.245 A  V1_T2=0.5 V  Tmeas2=125 C  EG_param=1  EG=1.11 eV  XTI_param=1  XTI=3  dBVdT=0 V/K  Tdevice=25 C  LocalVarLogging=[]  Rth=[ 0 10 ] K/W  thermal_mass_parameterization=1  thermal_mass=[ 0 1 ] J/K  thermal_time_constant=[ 0 10 ] s  thermal_mass_initial_temperatures=[ 25 25 ] C
  Inductor : fl_lib/Electrical/Electrical Elements/Inductor  l=2 H  i0=0 A  r=2 Ohm  g=1e-9 1/Ohm  i_Log=off  v_Log=off  i_L_Log=off  LocalVarNames=|i|v|i_L  LocalVarDescs=|i|v|Internal variable for current through inductor term  LocalVarLogging=[0 0 0]
  PS-Simulink Converter : nesl_utility/PS-Simulink Converter  PhysicalDomain=network_engine_domain  SubClassName=ps_output  LeftPortType=input  RightPortType=output  PseudoPeriodic=off  Frequencies=[]  Unit=1  AffineConversion=off
  PS-Simulink Converter1 : nesl_utility/PS-Simulink Converter  PhysicalDomain=network_engine_domain  SubClassName=ps_output  LeftPortType=input  RightPortType=output  PseudoPeriodic=off  Frequencies=[]  Unit=1  AffineConversion=off
  PS-Simulink Converter2 : nesl_utility/PS-Simulink Converter  PhysicalDomain=network_engine_domain  SubClassName=ps_output  LeftPortType=input  RightPortType=output  PseudoPeriodic=off  Frequencies=[]  Unit=1  AffineConversion=off
  A : PMIOPort  Port=1  Side=Left
  B : PMIOPort  Port=2  Side=Left
  C : PMIOPort  Port=3  Side=Left
  i_a : Outport
  i_b : Outport  Port=2
  i_c : Outport  Port=3
  wires:
  PS-Simulink Converter2/1 -> i_c/1
  PS-Simulink Converter1/1 -> i_b/1
  PS-Simulink Converter/1 -> i_a/1
  connections:
  Diode4/LConn1 -- Inductor/RConn1 -- Diode1/LConn1 -- Diode3/LConn1
  Diode5/LConn1 -- Current Sensor2/RConn2 -- Diode4/RConn1
  Diode3/RConn1 -- Current Sensor1/RConn2 -- Diode2/LConn1
  A/RConn1 -- Current Sensor/LConn1
  Diode5/RConn1 -- Inductor/LConn1 -- Diode2/RConn1 -- Diode/RConn1
  Diode1/RConn1 -- Diode/LConn1 -- Current Sensor/RConn2
  Current Sensor/RConn1 -- PS-Simulink Converter/LConn1
  Current Sensor2/RConn1 -- PS-Simulink Converter2/LConn1
  C/RConn1 -- Current Sensor2/LConn1
  B/RConn1 -- Current Sensor1/LConn1
  Current Sensor1/RConn1 -- PS-Simulink Converter1/LConn1
